simulink model "final_test2"  (Simulink 7.7)
settings: Solver=ode45  StartTime=0.0  StopTime=10.0  RelTol=1e-3
undefined symbols (not defined in the file): des_attributefunction_support, des_figposition
libraries: simeventsattributes2 x84, simeventsrouting1 x60, simeventsserver1 x31, commrandsrc2 x24, simeventsgenerators1 x16, simeventstranslate1 x15, simeventssink1 x12, simeventsqueue1 x8
(part 2 of 3)

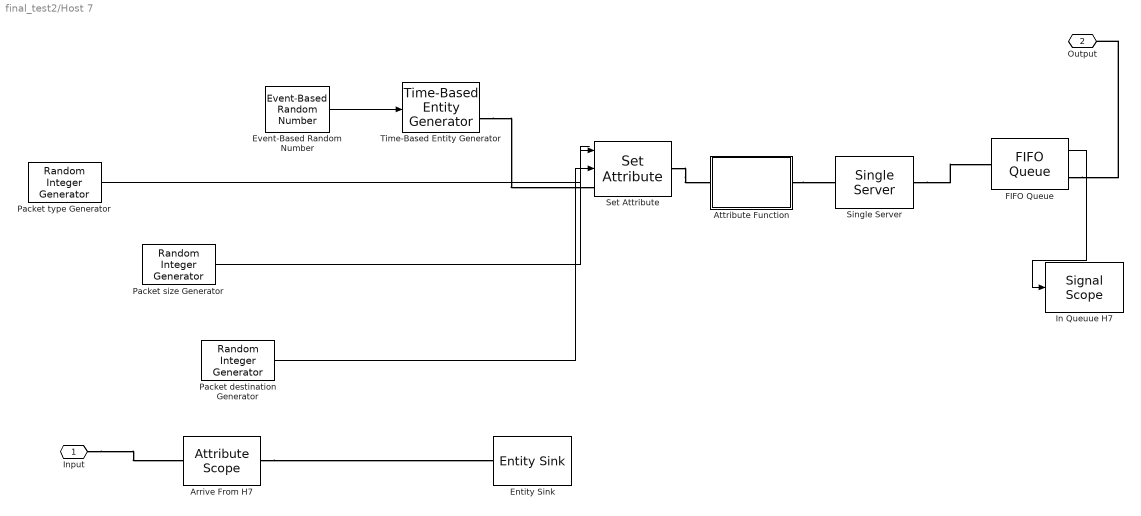
== system final_test2/Host 7 ==
  Arrive From H7 : simeventssink1/Attribute Scope  SystemSampleTime=-1  PlotType=Stair  InputType=Attribute  NumInputs=1  AttributeNameY=from  XInputOptionSignal=Event time  XInputOptionEntity=Event time  AttributeNameX=Count  EnableEntityOutport=on  XMin=0  XMax=10  XLimitExceededOption=Stretch axis limits  YLimitExceededOption=Stretch axis limits  AxisGrid=on  AxisLegend=off  LineDisables=""  LineColors=b  LineStyles=-  LineMarkers=.  OpenScopeAtSimStart=on  Title=""  YLabel=""  XLabel=Time  FigurePosition=des_figposition([5 25 25 25])  AxisZoom=off  DataStoreOption=Limited  DataPointsLimit=10000  StatNumberArrived=Off  ShowCountPlotted=off  ShowToolbar=on
      settings: YMin=0  YMax=10
  Attribute Function : Subsystem  LoadFcn=des_attributefunction_support(gcb,'LoadFcn');  StartFcn=des_attributefunction_support(gcb,'StartFcn');  mask(Attribute Function){OutputNamePrefix=out_}
      mask prompts: OutputNamePrefix "Prefix name"
      settings: CopyFcn=des_attributefunction_support(gcb,'CopyFcn');  OpenFcn=des_attributefunction_support(gcb,'OpenFcn');  ErrorFcn=des_error_redirect
      mask Help: helpview(simeventsbhelp('attributefunction'))
      mask Display: image(des_iconLoad('attribFunction.jpg'),'center');
  Entity Sink : simeventssink1/Entity Sink  SystemSampleTime=-1  AvailableForArrivals=on  StatNumberArrived=On
  Event-Based Random Number : simeventsgenerators1/Signal Generators/Event-Based Random Number  SystemSampleTime=-1  distribution=Poisson  meanExp=1  minUnif=1  maxUnif=1  pOneBern=0.25  pSuccessBino=0.5  numTrialBino=1  meanNorm=0  stdNorm=1  minTri=1  maxTri=3  modeTri=2  thresholdLogn=0  scaleLogn=1  shapeLogn=1  pSuccessGeo=0.5  meanPoiss=0.001  thresholdLogl=0  scaleLogl=1  thresholdGam=0  scaleGam=1  shapeGam=1  minBeta=0  maxBeta=1  shape1Beta=1  shape2Beta=1  minUnid=0  maxUnid=1  numValueUnid=2  thresholdWbl=0  scaleWbl=1  shapeWbl=1  valueVecCont=[0 1]  cdfVecCont=[0 1]  valueVecDisc=[0 1]  probVecDisc=[0.5 0.5]  seed=12345  IsProcessed=on  isConnected=1
  FIFO Queue : simeventsqueue1/FIFO Queue  SystemSampleTime=-1  Capacity=25  EnableTOPort=off  StatNumberDeparted=Off  StatNumberInBlock=On  StatPendingEntity=Off  StatAverageWait=Off  StatAverageQueueLength=Off  StatNumberTimedout=Off
  In Queuue H7 : simeventssink1/Signal Scope  SystemSampleTime=-1  PlotType=Stair  InputType=Signal  NumInputs=1  AttributeNameY=Count  XInputOptionSignal=Event time  XInputOptionEntity=Event time  AttributeNameX=Count  EnableEntityOutport=on  XMin=0  XMax=10  XLimitExceededOption=Stretch axis limits  YLimitExceededOption=Stretch axis limits  AxisGrid=on  AxisLegend=off  LineDisables=""  LineColors=b  LineStyles=-  LineMarkers=.  OpenScopeAtSimStart=on  Title=""  YLabel=""  XLabel=Time  FigurePosition=des_figposition([5 60 25 25])  AxisZoom=off  DataStoreOption=Limited  DataPointsLimit=10000  StatNumberArrived=Off  ShowCountPlotted=off  ShowToolbar=on
      settings: YMin=0  YMax=10
  Packet destination Generator : commrandsrc2/Random Integer Generator  SystemSampleTime=-1  mul=6  seed=22  Ts=1  frameBased=off  sampPerFrame=1  orient=off  outDataType=double
  Packet size Generator : commrandsrc2/Random Integer Generator  SystemSampleTime=-1  mul=2  seed=22  Ts=1  frameBased=off  sampPerFrame=1  orient=off  outDataType=double
  Packet type Generator : commrandsrc2/Random Integer Generator  SystemSampleTime=-1  mul=2  seed=37  Ts=1  frameBased=off  sampPerFrame=1  orient=off  outDataType=double
  Set Attribute : simeventsattributes2/Set Attribute  SystemSampleTime=-1  AttributeFrom=Dialog|Signal port|Signal port|Dialog  AttributeName=type|size|dest|from  AttributeTreatAsVector=1|1|1|1  AttributeValue=1|1|4|1  AttributeCreate=on  StatNumberDeparted=Off  EvaluatedAttributeValue={1;[];[];1}
  Single Server : simeventsserver1/Single Server  SystemSampleTime=-1  ServiceTimeFrom=Dialog  ServiceTime=0  AttributeName=ServiceTime  PriorityServiceCompletion=500  PermitPreemption=off  SortingAttributeName=PriorityAttributeName  SortingDirection=Ascending  WriteToAttribute=off  ResidualAttributeName=ResidualServiceTime  CreateAttribute=on  EnableTOPort=off  StatNumberDeparted=Off  StatNumberInBlock=Off  StatNumberPreempted=Off  StatPendingEntity=Off  StatAverageWait=Off  StatUtilization=Off  StatNumberTimedout=Off
  Time-Based Entity Generator : simeventsgenerators1/Entity Generators/Time-Based Entity Generator  SystemSampleTime=-1  GenerateEntitiesUpon=Intergeneration time from port t  Distribution=Constant  Minimum=0  Maximum=1  Mean=1  InitialSeed=12345  Period=1  PriorityEntityGeneration=300  GenerateEntityAtSimulationStart=on  ResponseWhenBlocked=Pause generation  ResponseWhenUnblocked=Immediate restart  EntityType=Standard  StatNumberDeparted=On  StatPendingEntity=Off  StatAverageIntergenerationTime=Off
  Input : PMIOPort  Port=1  Side=Right
  Output : PMIOPort  Port=2  Side=Right
  wires:
  Event-Based Random Number/1 -> Time-Based Entity Generator/1
  Packet size Generator/1 -> Set Attribute/1
  Packet type Generator/1 -> ?
  Packet destination Generator/1 -> Set Attribute/2
  FIFO Queue/1 -> In Queuue H7/1
  connections:
  Time-Based Entity Generator/RConn1 -- Set Attribute/LConn1
  Set Attribute/RConn1 -- Attribute Function/LConn1
  FIFO Queue/RConn1 -- Output/RConn1
  Attribute Function/RConn1 -- Single Server/LConn1
  Single Server/RConn1 -- FIFO Queue/LConn1
  Input/RConn1 -- Arrive From H7/LConn1
  Arrive From H7/RConn1 -- Entity Sink/LConn1

== system final_test2/Host 8 ==
  Attribute Function : Subsystem  LoadFcn=des_attributefunction_support(gcb,'LoadFcn');  StartFcn=des_attributefunction_support(gcb,'StartFcn');  mask(Attribute Function){OutputNamePrefix=out_}
      mask prompts: OutputNamePrefix "Prefix name"
      settings: CopyFcn=des_attributefunction_support(gcb,'CopyFcn');  OpenFcn=des_attributefunction_support(gcb,'OpenFcn');  ErrorFcn=des_error_redirect
      mask Help: helpview(simeventsbhelp('attributefunction'))
      mask Display: image(des_iconLoad('attribFunction.jpg'),'center');
  Entity Sink : simeventssink1/Entity Sink  SystemSampleTime=-1  AvailableForArrivals=on  StatNumberArrived=On
  Event-Based Random Number : simeventsgenerators1/Signal Generators/Event-Based Random Number  SystemSampleTime=-1  distribution=Poisson  meanExp=1  minUnif=1  maxUnif=1  pOneBern=0.25  pSuccessBino=0.5  numTrialBino=1  meanNorm=0  stdNorm=1  minTri=1  maxTri=3  modeTri=2  thresholdLogn=0  scaleLogn=1  shapeLogn=1  pSuccessGeo=0.5  meanPoiss=0.1  thresholdLogl=0  scaleLogl=1  thresholdGam=0  scaleGam=1  shapeGam=1  minBeta=0  maxBeta=1  shape1Beta=1  shape2Beta=1  minUnid=0  maxUnid=1  numValueUnid=2  thresholdWbl=0  scaleWbl=1  shapeWbl=1  valueVecCont=[0 1]  cdfVecCont=[0 1]  valueVecDisc=[0 1]  probVecDisc=[0.5 0.5]  seed=12345  IsProcessed=on  isConnected=1
  FIFO Queue : simeventsqueue1/FIFO Queue  SystemSampleTime=-1  Capacity=25  EnableTOPort=off  StatNumberDeparted=Off  StatNumberInBlock=Off  StatPendingEntity=Off  StatAverageWait=Off  StatAverageQueueLength=Off  StatNumberTimedout=Off
  Packet destination Generator : commrandsrc2/Random Integer Generator  SystemSampleTime=-1  mul=6  seed=22  Ts=1  frameBased=off  sampPerFrame=1  orient=off  outDataType=double
  Packet size Generator : commrandsrc2/Random Integer Generator  SystemSampleTime=-1  mul=2  seed=22  Ts=1  frameBased=off  sampPerFrame=1  orient=off  outDataType=double
  Packet type Generator : commrandsrc2/Random Integer Generator  SystemSampleTime=-1  mul=2  seed=37  Ts=1  frameBased=off  sampPerFrame=1  orient=off  outDataType=double
  Set Attribute : simeventsattributes2/Set Attribute  SystemSampleTime=-1  AttributeFrom=Signal port|Signal port|Signal port|Dialog  AttributeName=type|size|dest|from  AttributeTreatAsVector=1|1|1|1  AttributeValue=1|1|4|6  AttributeCreate=on  StatNumberDeparted=Off  EvaluatedAttributeValue={[];[];[];6}
  Single Server : simeventsserver1/Single Server  SystemSampleTime=-1  ServiceTimeFrom=Dialog  ServiceTime=0  AttributeName=ServiceTime  PriorityServiceCompletion=500  PermitPreemption=off  SortingAttributeName=PriorityAttributeName  SortingDirection=Ascending  WriteToAttribute=off  ResidualAttributeName=ResidualServiceTime  CreateAttribute=on  EnableTOPort=off  StatNumberDeparted=Off  StatNumberInBlock=Off  StatNumberPreempted=Off  StatPendingEntity=Off  StatAverageWait=Off  StatUtilization=Off  StatNumberTimedout=Off
  Time-Based Entity Generator : simeventsgenerators1/Entity Generators/Time-Based Entity Generator  SystemSampleTime=-1  GenerateEntitiesUpon=Intergeneration time from port t  Distribution=Constant  Minimum=0  Maximum=1  Mean=1  InitialSeed=12345  Period=1  PriorityEntityGeneration=300  GenerateEntityAtSimulationStart=on  ResponseWhenBlocked=Pause generation  ResponseWhenUnblocked=Immediate restart  EntityType=Standard  StatNumberDeparted=On  StatPendingEntity=Off  StatAverageIntergenerationTime=Off
  Input : PMIOPort  Port=1  Side=Left
  Output : PMIOPort  Port=2  Side=Left
  wires:
  Packet destination Generator/1 -> Set Attribute/3
  Packet type Generator/1 -> Set Attribute/1
  Packet size Generator/1 -> Set Attribute/2
  Event-Based Random Number/1 -> Time-Based Entity Generator/1
  connections:
  Single Server/RConn1 -- FIFO Queue/LConn1
  Attribute Function/RConn1 -- Single Server/LConn1
  FIFO Queue/RConn1 -- Output/RConn1
  Set Attribute/RConn1 -- Attribute Function/LConn1
  Input/RConn1 -- Entity Sink/LConn1
  Time-Based Entity Generator/RConn1 -- Set Attribute/LConn1

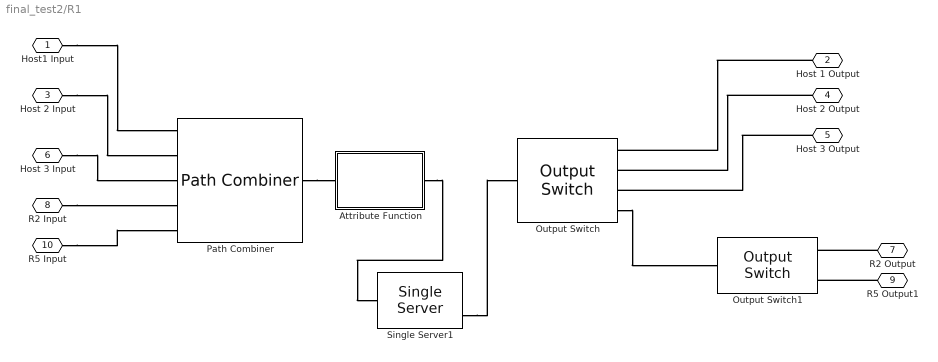
== system final_test2/R1 ==
  Attribute Function : Subsystem  LoadFcn=des_attributefunction_support(gcb,'LoadFcn');  StartFcn=des_attributefunction_support(gcb,'StartFcn');  mask(Attribute Function){OutputNamePrefix=out_}
      mask prompts: OutputNamePrefix "Prefix name"
      settings: CopyFcn=des_attributefunction_support(gcb,'CopyFcn');  OpenFcn=des_attributefunction_support(gcb,'OpenFcn');  ErrorFcn=des_error_redirect
      mask Help: helpview(simeventsbhelp('attributefunction'))
      mask Display: image(des_iconLoad('attribFunction.jpg'),'center');
  Output Switch : simeventsrouting1/Output Switch  SystemSampleTime=-1  NumberOutputPorts=4  SwitchingCriterion=From attribute  InitialSeed=34567  AttributeName=port  InitialConditionsOpt=off  InitialConditions=1  EntityBufferOpt=off  SpecifyEventPriority=off  PriorityOutputSwitchSelectPort=4100  TimeoutPortOpt=off  StatNumberDeparted=Off  StatNumberTimedOut=Off  StatPendingEntity=Off  StatLastDeparturePort=Off  EvaluatedNumPorts=4
  Output Switch1 : simeventsrouting1/Output Switch  SystemSampleTime=-1  NumberOutputPorts=2  SwitchingCriterion=First port that is not blocked  InitialSeed=34567  AttributeName=Attribute1  InitialConditionsOpt=off  InitialConditions=1  EntityBufferOpt=off  SpecifyEventPriority=off  PriorityOutputSwitchSelectPort=4100  TimeoutPortOpt=off  StatNumberDeparted=Off  StatNumberTimedOut=Off  StatPendingEntity=Off  StatLastDeparturePort=Off  EvaluatedNumPorts=2
  Path Combiner : simeventsrouting1/Path Combiner  SystemSampleTime=-1  NumberInputPorts=5  InputPortPrecedence=IN1 port  InitialSeed=45675  SpecifyEventPriority=off  PriorityPathCombinerPortPrecedenceSelection=4100  StatNumberDeparted=Off  StatLastArrivalPort=Off  EvaluatedNumPorts=5
  Single Server1 : simeventsserver1/Single Server  SystemSampleTime=-1  ServiceTimeFrom=Dialog  ServiceTime=0  AttributeName=ServiceTime  PriorityServiceCompletion=500  PermitPreemption=off  SortingAttributeName=PriorityAttributeName  SortingDirection=Ascending  WriteToAttribute=off  ResidualAttributeName=ResidualServiceTime  CreateAttribute=on  EnableTOPort=off  StatNumberDeparted=On  StatNumberInBlock=Off  StatNumberPreempted=Off  StatPendingEntity=Off  StatAverageWait=Off  StatUtilization=Off  StatNumberTimedout=Off
  Host1 Input : PMIOPort  Port=1  Side=Left
  Host 1 Output : PMIOPort  Port=2  Side=Left
  Host 2 Input : PMIOPort  Port=3  Side=Left
  Host 2 Output : PMIOPort  Port=4  Side=Left
  Host 3 Output : PMIOPort  Port=5  Side=Left
  Host 3 Input : PMIOPort  Port=6  Side=Left
  R2 Output : PMIOPort  Port=7  Side=Right
  R2 Input : PMIOPort  Port=8  Side=Right
  R5 Output1 : PMIOPort  Port=9  Side=Right
  R5 Input : PMIOPort  Port=10  Side=Right
  connections:
  Host 1 Output/RConn1 -- Output Switch/RConn1
  Host 2 Output/RConn1 -- Output Switch/RConn2
  Host 3 Output/RConn1 -- Output Switch/RConn3
  Host1 Input/RConn1 -- Path Combiner/LConn1
  Host 2 Input/RConn1 -- Path Combiner/LConn2
  Host 3 Input/RConn1 -- Path Combiner/LConn3
  R2 Input/RConn1 -- Path Combiner/LConn4
  R5 Input/RConn1 -- Path Combiner/LConn5
  Output Switch/RConn4 -- Output Switch1/LConn1
  R2 Output/RConn1 -- Output Switch1/RConn1
  R5 Output1/RConn1 -- Output Switch1/RConn2
  Path Combiner/RConn1 -- Attribute Function/LConn1
  Attribute Function/RConn1 -- Single Server1/LConn1
  Single Server1/RConn1 -- Output Switch/LConn1

== system final_test2/R2 ==
  Attribute Function : Subsystem  LoadFcn=des_attributefunction_support(gcb,'LoadFcn');  StartFcn=des_attributefunction_support(gcb,'StartFcn');  mask(Attribute Function){OutputNamePrefix=out_}
      mask prompts: OutputNamePrefix "Prefix name"
      settings: CopyFcn=des_attributefunction_support(gcb,'CopyFcn');  OpenFcn=des_attributefunction_support(gcb,'OpenFcn');  ErrorFcn=des_error_redirect
      mask Help: helpview(simeventsbhelp('attributefunction'))
      mask Display: image(des_iconLoad('attribFunction.jpg'),'center');
  Output Switch : simeventsrouting1/Output Switch  SystemSampleTime=-1  NumberOutputPorts=2  SwitchingCriterion=From attribute  InitialSeed=34567  AttributeName=port  InitialConditionsOpt=off  InitialConditions=1  EntityBufferOpt=off  SpecifyEventPriority=off  PriorityOutputSwitchSelectPort=4100  TimeoutPortOpt=off  StatNumberDeparted=Off  StatNumberTimedOut=Off  StatPendingEntity=Off  StatLastDeparturePort=Off  EvaluatedNumPorts=2
  Path Combiner : simeventsrouting1/Path Combiner  SystemSampleTime=-1  NumberInputPorts=2  InputPortPrecedence=IN1 port  InitialSeed=45675  SpecifyEventPriority=off  PriorityPathCombinerPortPrecedenceSelection=4100  StatNumberDeparted=Off  StatLastArrivalPort=Off  EvaluatedNumPorts=2
  Set Attribute : simeventsattributes2/Set Attribute  SystemSampleTime=-1  AttributeFrom=Dialog  AttributeName=rfrom  AttributeTreatAsVector=1  AttributeValue=1  AttributeCreate=on  StatNumberDeparted=Off  EvaluatedAttributeValue={1}
  Set Attribute1 : simeventsattributes2/Set Attribute  SystemSampleTime=-1  AttributeFrom=Dialog  AttributeName=rfrom  AttributeTreatAsVector=1  AttributeValue=3  AttributeCreate=on  StatNumberDeparted=Off  EvaluatedAttributeValue={3}
  Single Server : simeventsserver1/Single Server  SystemSampleTime=-1  ServiceTimeFrom=Dialog  ServiceTime=0  AttributeName=ServiceTime  PriorityServiceCompletion=500  PermitPreemption=off  SortingAttributeName=PriorityAttributeName  SortingDirection=Ascending  WriteToAttribute=off  ResidualAttributeName=ResidualServiceTime  CreateAttribute=on  EnableTOPort=off  StatNumberDeparted=Off  StatNumberInBlock=Off  StatNumberPreempted=Off  StatPendingEntity=Off  StatAverageWait=Off  StatUtilization=Off  StatNumberTimedout=Off
  R1 In : PMIOPort  Port=1  Side=Left
  R1 Out : PMIOPort  Port=2  Side=Left
  R3 Out : PMIOPort  Port=3  Side=Right
  R3 In : PMIOPort  Port=4  Side=Right
  connections:
  Path Combiner/RConn1 -- Attribute Function/LConn1
  Set Attribute/RConn1 -- Path Combiner/LConn1
  Set Attribute1/RConn1 -- Path Combiner/LConn2
  R1 In/RConn1 -- Set Attribute/LConn1
  R1 Out/RConn1 -- Output Switch/RConn1
  R3 Out/RConn1 -- Output Switch/RConn2
  R3 In/RConn1 -- Set Attribute1/LConn1
  Single Server/RConn1 -- Output Switch/LConn1
  Attribute Function/RConn1 -- Single Server/LConn1

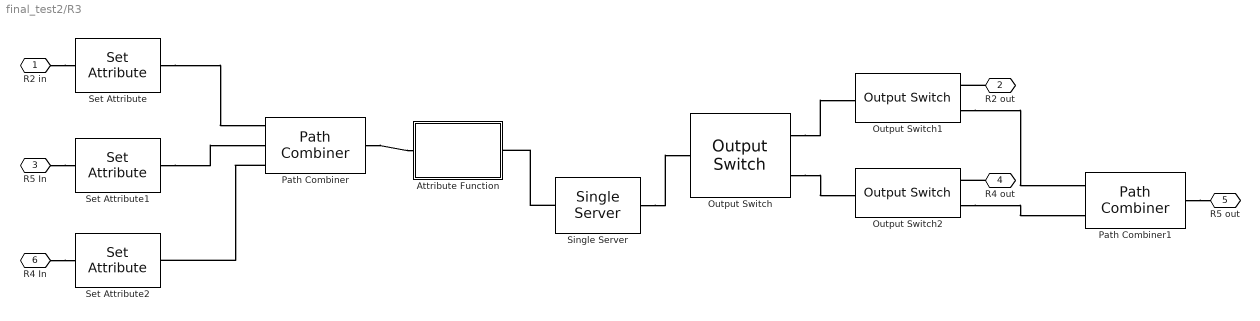
== system final_test2/R3 ==
  Attribute Function : Subsystem  LoadFcn=des_attributefunction_support(gcb,'LoadFcn');  StartFcn=des_attributefunction_support(gcb,'StartFcn');  mask(Attribute Function){OutputNamePrefix=out_}
      mask prompts: OutputNamePrefix "Prefix name"
      settings: CopyFcn=des_attributefunction_support(gcb,'CopyFcn');  OpenFcn=des_attributefunction_support(gcb,'OpenFcn');  ErrorFcn=des_error_redirect
      mask Help: helpview(simeventsbhelp('attributefunction'))
      mask Display: image(des_iconLoad('attribFunction.jpg'),'center');
  Output Switch : simeventsrouting1/Output Switch  SystemSampleTime=-1  NumberOutputPorts=2  SwitchingCriterion=From attribute  InitialSeed=34567  AttributeName=port  InitialConditionsOpt=off  InitialConditions=1  EntityBufferOpt=off  SpecifyEventPriority=off  PriorityOutputSwitchSelectPort=4100  TimeoutPortOpt=off  StatNumberDeparted=Off  StatNumberTimedOut=Off  StatPendingEntity=Off  StatLastDeparturePort=Off  EvaluatedNumPorts=2
  Output Switch1 : simeventsrouting1/Output Switch  SystemSampleTime=-1  NumberOutputPorts=2  SwitchingCriterion=First port that is not blocked  InitialSeed=34567  AttributeName=port  InitialConditionsOpt=off  InitialConditions=1  EntityBufferOpt=off  SpecifyEventPriority=off  PriorityOutputSwitchSelectPort=4100  TimeoutPortOpt=off  StatNumberDeparted=Off  StatNumberTimedOut=Off  StatPendingEntity=Off  StatLastDeparturePort=Off  EvaluatedNumPorts=2
  Output Switch2 : simeventsrouting1/Output Switch  SystemSampleTime=-1  NumberOutputPorts=2  SwitchingCriterion=First port that is not blocked  InitialSeed=34567  AttributeName=port  InitialConditionsOpt=off  InitialConditions=1  EntityBufferOpt=off  SpecifyEventPriority=off  PriorityOutputSwitchSelectPort=4100  TimeoutPortOpt=off  StatNumberDeparted=Off  StatNumberTimedOut=Off  StatPendingEntity=Off  StatLastDeparturePort=Off  EvaluatedNumPorts=2
  Path Combiner : simeventsrouting1/Path Combiner  SystemSampleTime=-1  NumberInputPorts=3  InputPortPrecedence=IN1 port  InitialSeed=45675  SpecifyEventPriority=off  PriorityPathCombinerPortPrecedenceSelection=4100  StatNumberDeparted=Off  StatLastArrivalPort=Off  EvaluatedNumPorts=3
  Path Combiner1 : simeventsrouting1/Path Combiner  SystemSampleTime=-1  NumberInputPorts=2  InputPortPrecedence=IN1 port  InitialSeed=45675  SpecifyEventPriority=off  PriorityPathCombinerPortPrecedenceSelection=4100  StatNumberDeparted=Off  StatLastArrivalPort=Off  EvaluatedNumPorts=2
  Set Attribute : simeventsattributes2/Set Attribute  SystemSampleTime=-1  AttributeFrom=Dialog  AttributeName=rfrom  AttributeTreatAsVector=1  AttributeValue=2  AttributeCreate=on  StatNumberDeparted=Off  EvaluatedAttributeValue={2}
  Set Attribute1 : simeventsattributes2/Set Attribute  SystemSampleTime=-1  AttributeFrom=Dialog  AttributeName=rfrom  AttributeTreatAsVector=1  AttributeValue=5  AttributeCreate=on  StatNumberDeparted=Off  EvaluatedAttributeValue={5}
  Set Attribute2 : simeventsattributes2/Set Attribute  SystemSampleTime=-1  AttributeFrom=Dialog  AttributeName=rfrom  AttributeTreatAsVector=1  AttributeValue=4  AttributeCreate=on  StatNumberDeparted=Off  EvaluatedAttributeValue={4}
  Single Server : simeventsserver1/Single Server  SystemSampleTime=-1  ServiceTimeFrom=Dialog  ServiceTime=0  AttributeName=ServiceTime  PriorityServiceCompletion=500  PermitPreemption=off  SortingAttributeName=PriorityAttributeName  SortingDirection=Ascending  WriteToAttribute=off  ResidualAttributeName=ResidualServiceTime  CreateAttribute=on  EnableTOPort=off  StatNumberDeparted=Off  StatNumberInBlock=Off  StatNumberPreempted=Off  StatPendingEntity=Off  StatAverageWait=Off  StatUtilization=Off  StatNumberTimedout=Off
  R2 in : PMIOPort  Port=1  Side=Left
  R2 out : PMIOPort  Port=2  Side=Left
  R5 In : PMIOPort  Port=3  Side=Left
  R4 out : PMIOPort  Port=4  Side=Right
  R5 out : PMIOPort  Port=5  Side=Left
  R4 In : PMIOPort  Port=6  Side=Right
  connections:
  Path Combiner/RConn1 -- Attribute Function/LConn1
  Output Switch/RConn1 -- Output Switch1/LConn1
  Output Switch/RConn2 -- Output Switch2/LConn1
  Set Attribute/RConn1 -- Path Combiner/LConn1
  Set Attribute1/RConn1 -- Path Combiner/LConn2
  Path Combiner/LConn3 -- Set Attribute2/RConn1
  R2 in/RConn1 -- Set Attribute/LConn1
  R2 out/RConn1 -- Output Switch1/RConn1
  R5 In/RConn1 -- Set Attribute1/LConn1
  R4 out/RConn1 -- Output Switch2/RConn1
  R4 In/RConn1 -- Set Attribute2/LConn1
  Path Combiner1/RConn1 -- R5 out/RConn1
  Output Switch2/RConn2 -- Path Combiner1/LConn2
  Output Switch1/RConn2 -- Path Combiner1/LConn1
  Single Server/RConn1 -- Output Switch/LConn1
  Single Server/LConn1 -- Attribute Function/RConn1

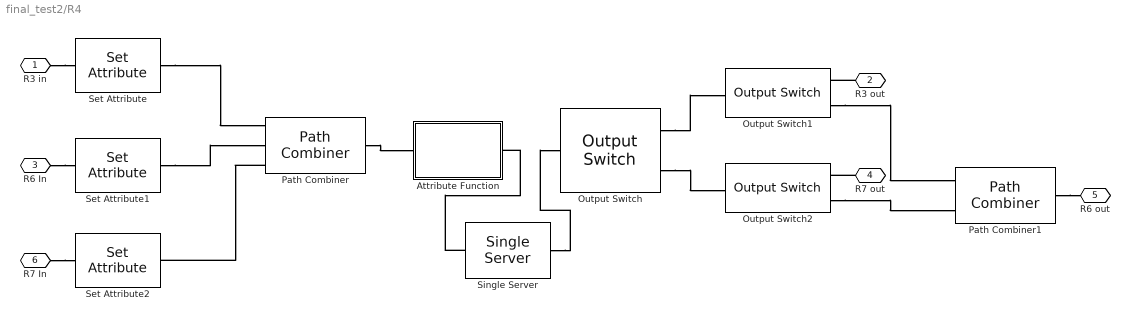
== system final_test2/R4 ==
  Attribute Function : Subsystem  LoadFcn=des_attributefunction_support(gcb,'LoadFcn');  StartFcn=des_attributefunction_support(gcb,'StartFcn');  mask(Attribute Function){OutputNamePrefix=out_}
      mask prompts: OutputNamePrefix "Prefix name"
      settings: CopyFcn=des_attributefunction_support(gcb,'CopyFcn');  OpenFcn=des_attributefunction_support(gcb,'OpenFcn');  ErrorFcn=des_error_redirect
      mask Help: helpview(simeventsbhelp('attributefunction'))
      mask Display: image(des_iconLoad('attribFunction.jpg'),'center');
  Output Switch : simeventsrouting1/Output Switch  SystemSampleTime=-1  NumberOutputPorts=2  SwitchingCriterion=From attribute  InitialSeed=34567  AttributeName=port  InitialConditionsOpt=off  InitialConditions=1  EntityBufferOpt=off  SpecifyEventPriority=off  PriorityOutputSwitchSelectPort=4100  TimeoutPortOpt=off  StatNumberDeparted=Off  StatNumberTimedOut=Off  StatPendingEntity=Off  StatLastDeparturePort=Off  EvaluatedNumPorts=2
  Output Switch1 : simeventsrouting1/Output Switch  SystemSampleTime=-1  NumberOutputPorts=2  SwitchingCriterion=First port that is not blocked  InitialSeed=34567  AttributeName=port  InitialConditionsOpt=off  InitialConditions=1  EntityBufferOpt=off  SpecifyEventPriority=off  PriorityOutputSwitchSelectPort=4100  TimeoutPortOpt=off  StatNumberDeparted=Off  StatNumberTimedOut=Off  StatPendingEntity=Off  StatLastDeparturePort=Off  EvaluatedNumPorts=2
  Output Switch2 : simeventsrouting1/Output Switch  SystemSampleTime=-1  NumberOutputPorts=2  SwitchingCriterion=First port that is not blocked  InitialSeed=34567  AttributeName=port  InitialConditionsOpt=off  InitialConditions=1  EntityBufferOpt=off  SpecifyEventPriority=off  PriorityOutputSwitchSelectPort=4100  TimeoutPortOpt=off  StatNumberDeparted=Off  StatNumberTimedOut=Off  StatPendingEntity=Off  StatLastDeparturePort=Off  EvaluatedNumPorts=2
  Path Combiner : simeventsrouting1/Path Combiner  SystemSampleTime=-1  NumberInputPorts=3  InputPortPrecedence=IN1 port  InitialSeed=45675  SpecifyEventPriority=off  PriorityPathCombinerPortPrecedenceSelection=4100  StatNumberDeparted=Off  StatLastArrivalPort=Off  EvaluatedNumPorts=3
  Path Combiner1 : simeventsrouting1/Path Combiner  SystemSampleTime=-1  NumberInputPorts=2  InputPortPrecedence=IN1 port  InitialSeed=45675  SpecifyEventPriority=off  PriorityPathCombinerPortPrecedenceSelection=4100  StatNumberDeparted=Off  StatLastArrivalPort=Off  EvaluatedNumPorts=2
  Set Attribute : simeventsattributes2/Set Attribute  SystemSampleTime=-1  AttributeFrom=Dialog  AttributeName=rfrom  AttributeTreatAsVector=1  AttributeValue=3  AttributeCreate=on  StatNumberDeparted=Off  EvaluatedAttributeValue={3}
  Set Attribute1 : simeventsattributes2/Set Attribute  SystemSampleTime=-1  AttributeFrom=Dialog  AttributeName=rfrom  AttributeTreatAsVector=1  AttributeValue=6  AttributeCreate=on  StatNumberDeparted=Off  EvaluatedAttributeValue={6}
  Set Attribute2 : simeventsattributes2/Set Attribute  SystemSampleTime=-1  AttributeFrom=Dialog  AttributeName=rfrom  AttributeTreatAsVector=1  AttributeValue=7  AttributeCreate=on  StatNumberDeparted=Off  EvaluatedAttributeValue={7}
  Single Server : simeventsserver1/Single Server  SystemSampleTime=-1  ServiceTimeFrom=Dialog  ServiceTime=0  AttributeName=ServiceTime  PriorityServiceCompletion=500  PermitPreemption=off  SortingAttributeName=PriorityAttributeName  SortingDirection=Ascending  WriteToAttribute=off  ResidualAttributeName=ResidualServiceTime  CreateAttribute=on  EnableTOPort=off  StatNumberDeparted=Off  StatNumberInBlock=Off  StatNumberPreempted=Off  StatPendingEntity=Off  StatAverageWait=Off  StatUtilization=Off  StatNumberTimedout=Off
  R3 in : PMIOPort  Port=1  Side=Left
  R3 out : PMIOPort  Port=2  Side=Left
  R6 In : PMIOPort  Port=3  Side=Left
  R7 out : PMIOPort  Port=4  Side=Right
  R6 out : PMIOPort  Port=5  Side=Left
  R7 In : PMIOPort  Port=6  Side=Right
  connections:
  Output Switch1/RConn2 -- Path Combiner1/LConn1
  Output Switch2/RConn2 -- Path Combiner1/LConn2
  Path Combiner1/RConn1 -- R6 out/RConn1
  R7 In/RConn1 -- Set Attribute2/LConn1
  R7 out/RConn1 -- Output Switch2/RConn1
  R6 In/RConn1 -- Set Attribute1/LConn1
  R3 out/RConn1 -- Output Switch1/RConn1
  R3 in/RConn1 -- Set Attribute/LConn1
  Path Combiner/LConn3 -- Set Attribute2/RConn1
  Set Attribute1/RConn1 -- Path Combiner/LConn2
  Set Attribute/RConn1 -- Path Combiner/LConn1
  Output Switch/RConn2 -- Output Switch2/LConn1
  Output Switch/RConn1 -- Output Switch1/LConn1
  Path Combiner/RConn1 -- Attribute Function/LConn1
  Single Server/LConn1 -- Attribute Function/RConn1
  Single Server/RConn1 -- Output Switch/LConn1

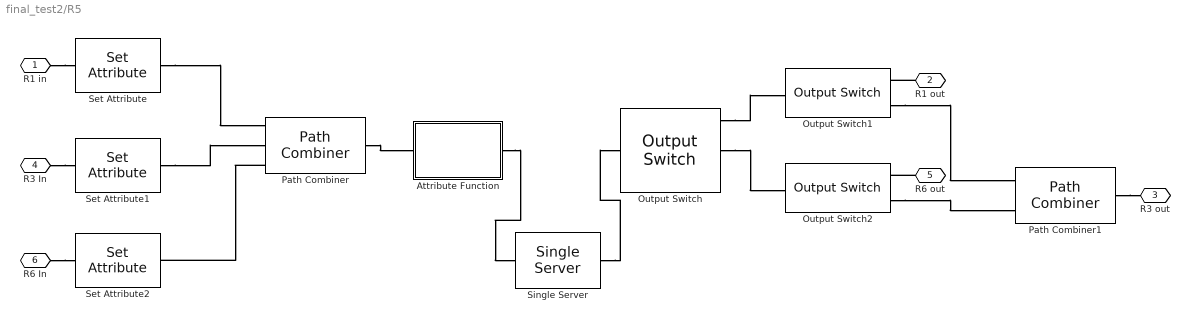
== system final_test2/R5 ==
  Attribute Function : Subsystem  LoadFcn=des_attributefunction_support(gcb,'LoadFcn');  StartFcn=des_attributefunction_support(gcb,'StartFcn');  mask(Attribute Function){OutputNamePrefix=out_}
      mask prompts: OutputNamePrefix "Prefix name"
      settings: CopyFcn=des_attributefunction_support(gcb,'CopyFcn');  OpenFcn=des_attributefunction_support(gcb,'OpenFcn');  ErrorFcn=des_error_redirect
      mask Help: helpview(simeventsbhelp('attributefunction'))
      mask Display: image(des_iconLoad('attribFunction.jpg'),'center');
  Output Switch : simeventsrouting1/Output Switch  SystemSampleTime=-1  NumberOutputPorts=3  SwitchingCriterion=From attribute  InitialSeed=34567  AttributeName=port  InitialConditionsOpt=off  InitialConditions=1  EntityBufferOpt=off  SpecifyEventPriority=off  PriorityOutputSwitchSelectPort=4100  TimeoutPortOpt=off  StatNumberDeparted=Off  StatNumberTimedOut=Off  StatPendingEntity=Off  StatLastDeparturePort=Off  EvaluatedNumPorts=3
  Output Switch1 : simeventsrouting1/Output Switch  SystemSampleTime=-1  NumberOutputPorts=2  SwitchingCriterion=First port that is not blocked  InitialSeed=34567  AttributeName=port  InitialConditionsOpt=off  InitialConditions=1  EntityBufferOpt=off  SpecifyEventPriority=off  PriorityOutputSwitchSelectPort=4100  TimeoutPortOpt=off  StatNumberDeparted=Off  StatNumberTimedOut=Off  StatPendingEntity=Off  StatLastDeparturePort=Off  EvaluatedNumPorts=2
  Output Switch2 : simeventsrouting1/Output Switch  SystemSampleTime=-1  NumberOutputPorts=2  SwitchingCriterion=First port that is not blocked  InitialSeed=34567  AttributeName=port  InitialConditionsOpt=off  InitialConditions=1  EntityBufferOpt=off  SpecifyEventPriority=off  PriorityOutputSwitchSelectPort=4100  TimeoutPortOpt=off  StatNumberDeparted=Off  StatNumberTimedOut=Off  StatPendingEntity=Off  StatLastDeparturePort=Off  EvaluatedNumPorts=2
  Path Combiner : simeventsrouting1/Path Combiner  SystemSampleTime=-1  NumberInputPorts=3  InputPortPrecedence=IN1 port  InitialSeed=45675  SpecifyEventPriority=off  PriorityPathCombinerPortPrecedenceSelection=4100  StatNumberDeparted=Off  StatLastArrivalPort=Off  EvaluatedNumPorts=3
  Path Combiner1 : simeventsrouting1/Path Combiner  SystemSampleTime=-1  NumberInputPorts=2  InputPortPrecedence=IN1 port  InitialSeed=45675  SpecifyEventPriority=off  PriorityPathCombinerPortPrecedenceSelection=4100  StatNumberDeparted=Off  StatLastArrivalPort=Off  EvaluatedNumPorts=2
  Set Attribute : simeventsattributes2/Set Attribute  SystemSampleTime=-1  AttributeFrom=Dialog  AttributeName=rfrom  AttributeTreatAsVector=1  AttributeValue=1  AttributeCreate=on  StatNumberDeparted=Off  EvaluatedAttributeValue={1}
  Set Attribute1 : simeventsattributes2/Set Attribute  SystemSampleTime=-1  AttributeFrom=Dialog  AttributeName=rfrom  AttributeTreatAsVector=1  AttributeValue=3  AttributeCreate=on  StatNumberDeparted=Off  EvaluatedAttributeValue={3}
  Set Attribute2 : simeventsattributes2/Set Attribute  SystemSampleTime=-1  AttributeFrom=Dialog  AttributeName=rfrom  AttributeTreatAsVector=1  AttributeValue=6  AttributeCreate=on  StatNumberDeparted=Off  EvaluatedAttributeValue={6}
  Single Server : simeventsserver1/Single Server  SystemSampleTime=-1  ServiceTimeFrom=Dialog  ServiceTime=0  AttributeName=ServiceTime  PriorityServiceCompletion=500  PermitPreemption=off  SortingAttributeName=PriorityAttributeName  SortingDirection=Ascending  WriteToAttribute=off  ResidualAttributeName=ResidualServiceTime  CreateAttribute=on  EnableTOPort=off  StatNumberDeparted=Off  StatNumberInBlock=Off  StatNumberPreempted=Off  StatPendingEntity=Off  StatAverageWait=Off  StatUtilization=Off  StatNumberTimedout=Off
  R1 in : PMIOPort  Port=1  Side=Left
  R1 out : PMIOPort  Port=2  Side=Left
  R3 out : PMIOPort  Port=3  Side=Right
  R3 In : PMIOPort  Port=4  Side=Right
  R6 out : PMIOPort  Port=5  Side=Right
  R6 In : PMIOPort  Port=6  Side=Right
  connections:
  Output Switch1/RConn2 -- Path Combiner1/LConn1
  Output Switch2/RConn2 -- Path Combiner1/LConn2
  Path Combiner1/RConn1 -- R3 out/RConn1
  R6 In/RConn1 -- Set Attribute2/LConn1
  R6 out/RConn1 -- Output Switch2/RConn1
  R3 In/RConn1 -- Set Attribute1/LConn1
  R1 out/RConn1 -- Output Switch1/RConn1
  R1 in/RConn1 -- Set Attribute/LConn1
  Path Combiner/LConn3 -- Set Attribute2/RConn1
  Set Attribute1/RConn1 -- Path Combiner/LConn2
  Set Attribute/RConn1 -- Path Combiner/LConn1
  Path Combiner/RConn1 -- Attribute Function/LConn1
  Output Switch/RConn1 -- Output Switch1/LConn1
  Output Switch/RConn2 -- Output Switch2/LConn1
  Attribute Function/RConn1 -- Single Server/LConn1
  Single Server/RConn1 -- Output Switch/LConn1

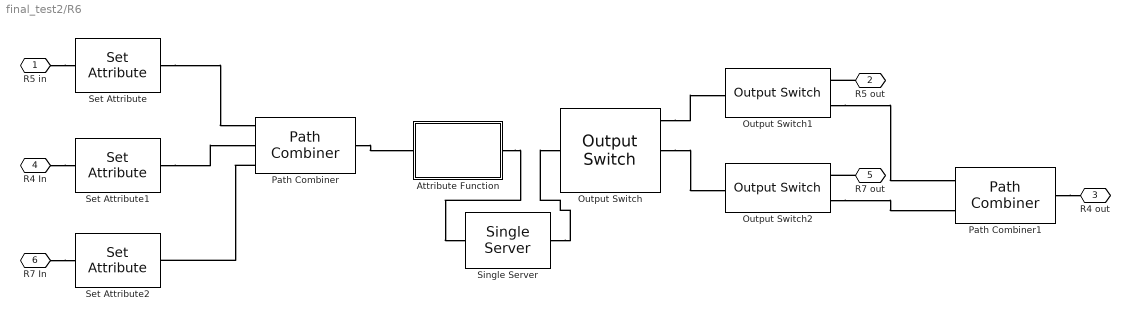
== system final_test2/R6 ==
  Attribute Function : Subsystem  LoadFcn=des_attributefunction_support(gcb,'LoadFcn');  StartFcn=des_attributefunction_support(gcb,'StartFcn');  mask(Attribute Function){OutputNamePrefix=out_}
      mask prompts: OutputNamePrefix "Prefix name"
      settings: CopyFcn=des_attributefunction_support(gcb,'CopyFcn');  OpenFcn=des_attributefunction_support(gcb,'OpenFcn');  ErrorFcn=des_error_redirect
      mask Help: helpview(simeventsbhelp('attributefunction'))
      mask Display: image(des_iconLoad('attribFunction.jpg'),'center');
  Output Switch : simeventsrouting1/Output Switch  SystemSampleTime=-1  NumberOutputPorts=3  SwitchingCriterion=From attribute  InitialSeed=34567  AttributeName=port  InitialConditionsOpt=off  InitialConditions=1  EntityBufferOpt=off  SpecifyEventPriority=off  PriorityOutputSwitchSelectPort=4100  TimeoutPortOpt=off  StatNumberDeparted=Off  StatNumberTimedOut=Off  StatPendingEntity=Off  StatLastDeparturePort=Off  EvaluatedNumPorts=3
  Output Switch1 : simeventsrouting1/Output Switch  SystemSampleTime=-1  NumberOutputPorts=2  SwitchingCriterion=First port that is not blocked  InitialSeed=34567  AttributeName=port  InitialConditionsOpt=off  InitialConditions=1  EntityBufferOpt=off  SpecifyEventPriority=off  PriorityOutputSwitchSelectPort=4100  TimeoutPortOpt=off  StatNumberDeparted=Off  StatNumberTimedOut=Off  StatPendingEntity=Off  StatLastDeparturePort=Off  EvaluatedNumPorts=2
  Output Switch2 : simeventsrouting1/Output Switch  SystemSampleTime=-1  NumberOutputPorts=2  SwitchingCriterion=First port that is not blocked  InitialSeed=34567  AttributeName=port  InitialConditionsOpt=off  InitialConditions=1  EntityBufferOpt=off  SpecifyEventPriority=off  PriorityOutputSwitchSelectPort=4100  TimeoutPortOpt=off  StatNumberDeparted=Off  StatNumberTimedOut=Off  StatPendingEntity=Off  StatLastDeparturePort=Off  EvaluatedNumPorts=2
  Path Combiner : simeventsrouting1/Path Combiner  SystemSampleTime=-1  NumberInputPorts=3  InputPortPrecedence=IN1 port  InitialSeed=45675  SpecifyEventPriority=off  PriorityPathCombinerPortPrecedenceSelection=4100  StatNumberDeparted=Off  StatLastArrivalPort=Off  EvaluatedNumPorts=3
  Path Combiner1 : simeventsrouting1/Path Combiner  SystemSampleTime=-1  NumberInputPorts=2  InputPortPrecedence=IN1 port  InitialSeed=45675  SpecifyEventPriority=off  PriorityPathCombinerPortPrecedenceSelection=4100  StatNumberDeparted=Off  StatLastArrivalPort=Off  EvaluatedNumPorts=2
  Set Attribute : simeventsattributes2/Set Attribute  SystemSampleTime=-1  AttributeFrom=Dialog  AttributeName=rfrom  AttributeTreatAsVector=1  AttributeValue=5  AttributeCreate=on  StatNumberDeparted=Off  EvaluatedAttributeValue={5}
  Set Attribute1 : simeventsattributes2/Set Attribute  SystemSampleTime=-1  AttributeFrom=Dialog  AttributeName=rfrom  AttributeTreatAsVector=1  AttributeValue=4  AttributeCreate=on  StatNumberDeparted=Off  EvaluatedAttributeValue={4}
  Set Attribute2 : simeventsattributes2/Set Attribute  SystemSampleTime=-1  AttributeFrom=Dialog  AttributeName=rfrom  AttributeTreatAsVector=1  AttributeValue=5  AttributeCreate=on  StatNumberDeparted=Off  EvaluatedAttributeValue={5}
  Single Server : simeventsserver1/Single Server  SystemSampleTime=-1  ServiceTimeFrom=Dialog  ServiceTime=0  AttributeName=ServiceTime  PriorityServiceCompletion=500  PermitPreemption=off  SortingAttributeName=PriorityAttributeName  SortingDirection=Ascending  WriteToAttribute=off  ResidualAttributeName=ResidualServiceTime  CreateAttribute=on  EnableTOPort=off  StatNumberDeparted=Off  StatNumberInBlock=Off  StatNumberPreempted=Off  StatPendingEntity=Off  StatAverageWait=Off  StatUtilization=Off  StatNumberTimedout=Off
  R5 in : PMIOPort  Port=1  Side=Left
  R5 out : PMIOPort  Port=2  Side=Left
  R4 out : PMIOPort  Port=3  Side=Right
  R4 In : PMIOPort  Port=4  Side=Right
  R7 out : PMIOPort  Port=5  Side=Right
  R7 In : PMIOPort  Port=6  Side=Right
  connections:
  Output Switch/RConn2 -- Output Switch2/LConn1
  Output Switch/RConn1 -- Output Switch1/LConn1
  Path Combiner/RConn1 -- Attribute Function/LConn1
  Set Attribute/RConn1 -- Path Combiner/LConn1
  Set Attribute1/RConn1 -- Path Combiner/LConn2
  Path Combiner/LConn3 -- Set Attribute2/RConn1
  R5 in/RConn1 -- Set Attribute/LConn1
  R5 out/RConn1 -- Output Switch1/RConn1
  R4 In/RConn1 -- Set Attribute1/LConn1
  R7 out/RConn1 -- Output Switch2/RConn1
  R7 In/RConn1 -- Set Attribute2/LConn1
  Path Combiner1/RConn1 -- R4 out/RConn1
  Output Switch2/RConn2 -- Path Combiner1/LConn2
  Output Switch1/RConn2 -- Path Combiner1/LConn1
  Attribute Function/RConn1 -- Single Server/LConn1
  Single Server/RConn1 -- Output Switch/LConn1

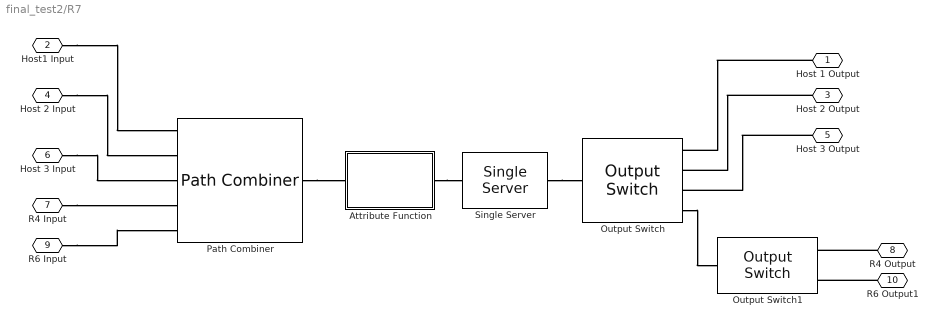
== system final_test2/R7 ==
  Attribute Function : Subsystem  LoadFcn=des_attributefunction_support(gcb,'LoadFcn');  StartFcn=des_attributefunction_support(gcb,'StartFcn');  mask(Attribute Function){OutputNamePrefix=out_}
      mask prompts: OutputNamePrefix "Prefix name"
      settings: CopyFcn=des_attributefunction_support(gcb,'CopyFcn');  OpenFcn=des_attributefunction_support(gcb,'OpenFcn');  ErrorFcn=des_error_redirect
      mask Help: helpview(simeventsbhelp('attributefunction'))
      mask Display: image(des_iconLoad('attribFunction.jpg'),'center');
  Output Switch : simeventsrouting1/Output Switch  SystemSampleTime=-1  NumberOutputPorts=4  SwitchingCriterion=From attribute  InitialSeed=34567  AttributeName=port  InitialConditionsOpt=off  InitialConditions=1  EntityBufferOpt=off  SpecifyEventPriority=off  PriorityOutputSwitchSelectPort=4100  TimeoutPortOpt=off  StatNumberDeparted=Off  StatNumberTimedOut=Off  StatPendingEntity=Off  StatLastDeparturePort=Off  EvaluatedNumPorts=4
  Output Switch1 : simeventsrouting1/Output Switch  SystemSampleTime=-1  NumberOutputPorts=2  SwitchingCriterion=First port that is not blocked  InitialSeed=34567  AttributeName=Attribute1  InitialConditionsOpt=off  InitialConditions=1  EntityBufferOpt=off  SpecifyEventPriority=off  PriorityOutputSwitchSelectPort=4100  TimeoutPortOpt=off  StatNumberDeparted=Off  StatNumberTimedOut=Off  StatPendingEntity=Off  StatLastDeparturePort=Off  EvaluatedNumPorts=2
  Path Combiner : simeventsrouting1/Path Combiner  SystemSampleTime=-1  NumberInputPorts=5  InputPortPrecedence=IN1 port  InitialSeed=45675  SpecifyEventPriority=off  PriorityPathCombinerPortPrecedenceSelection=4100  StatNumberDeparted=Off  StatLastArrivalPort=Off  EvaluatedNumPorts=5
  Single Server : simeventsserver1/Single Server  SystemSampleTime=-1  ServiceTimeFrom=Dialog  ServiceTime=0  AttributeName=ServiceTime  PriorityServiceCompletion=500  PermitPreemption=off  SortingAttributeName=PriorityAttributeName  SortingDirection=Ascending  WriteToAttribute=off  ResidualAttributeName=ResidualServiceTime  CreateAttribute=on  EnableTOPort=off  StatNumberDeparted=Off  StatNumberInBlock=Off  StatNumberPreempted=Off  StatPendingEntity=Off  StatAverageWait=Off  StatUtilization=Off  StatNumberTimedout=Off
  Host 1 Output : PMIOPort  Port=1  Side=Right
  Host1 Input : PMIOPort  Port=2  Side=Right
  Host 2 Output : PMIOPort  Port=3  Side=Right
  Host 2 Input : PMIOPort  Port=4  Side=Right
  Host 3 Output : PMIOPort  Port=5  Side=Right
  Host 3 Input : PMIOPort  Port=6  Side=Right
  R4 Input : PMIOPort  Port=7  Side=Left
  R4 Output : PMIOPort  Port=8  Side=Left
  R6 Input : PMIOPort  Port=9  Side=Left
  R6 Output1 : PMIOPort  Port=10  Side=Left
  connections:
  Single Server/RConn1 -- Output Switch/LConn1
  Attribute Function/RConn1 -- Single Server/LConn1
  R6 Output1/RConn1 -- Output Switch1/RConn2
  R4 Output/RConn1 -- Output Switch1/RConn1
  Output Switch/RConn4 -- Output Switch1/LConn1
  R6 Input/RConn1 -- Path Combiner/LConn5
  R4 Input/RConn1 -- Path Combiner/LConn4
  Host 3 Input/RConn1 -- Path Combiner/LConn3
  Host 2 Input/RConn1 -- Path Combiner/LConn2
  Host1 Input/RConn1 -- Path Combiner/LConn1
  Host 3 Output/RConn1 -- Output Switch/RConn3
  Host 2 Output/RConn1 -- Output Switch/RConn2
  Host 1 Output/RConn1 -- Output Switch/RConn1
  Path Combiner/RConn1 -- Attribute Function/LConn1

== system final_test2/Red Link ==
  N-Server : simeventsserver1/N-Server  SystemSampleTime=-1  NumberOfServers=2  ServiceTimeFrom=Dialog  ServiceTime=0.001  AttributeName=ServiceTime  PriorityServiceCompletion=500  EnableTOPort=off  StatNumberDeparted=Off  StatNumberInBlock=Off  StatPendingEntity=Off  StatNumberPending=Off  StatAverageWait=Off  StatUtilization=Off  StatNumberTimedout=Off
  Output Switch : simeventsrouting1/Output Switch  SystemSampleTime=-1  NumberOutputPorts=2  SwitchingCriterion=From attribute  InitialSeed=34567  AttributeName=port  InitialConditionsOpt=off  InitialConditions=1  EntityBufferOpt=off  SpecifyEventPriority=off  PriorityOutputSwitchSelectPort=4100  TimeoutPortOpt=off  StatNumberDeparted=Off  StatNumberTimedOut=Off  StatPendingEntity=Off  StatLastDeparturePort=Off  EvaluatedNumPorts=2
  Path Combiner : simeventsrouting1/Path Combiner  SystemSampleTime=-1  NumberInputPorts=2  InputPortPrecedence=IN1 port  InitialSeed=45675  SpecifyEventPriority=off  PriorityPathCombinerPortPrecedenceSelection=4100  StatNumberDeparted=Off  StatLastArrivalPort=Off  EvaluatedNumPorts=2
  Set Attribute : simeventsattributes2/Set Attribute  SystemSampleTime=-1  AttributeFrom=Dialog  AttributeName=port  AttributeTreatAsVector=1  AttributeValue=1  AttributeCreate=on  StatNumberDeparted=Off  EvaluatedAttributeValue={1}
  Set Attribute1 : simeventsattributes2/Set Attribute  SystemSampleTime=-1  AttributeFrom=Dialog  AttributeName=port  AttributeTreatAsVector=1  AttributeValue=2  AttributeCreate=on  StatNumberDeparted=Off  EvaluatedAttributeValue={2}
  Input1 : PMIOPort  Port=1  Side=Left
  Output1 : PMIOPort  Port=2  Side=Right
  Input2 : PMIOPort  Port=3  Side=Right
  Output2 : PMIOPort  Port=4  Side=Left
  connections:
  Path Combiner/RConn1 -- N-Server/LConn1
  N-Server/RConn1 -- Output Switch/LConn1
  Output Switch/RConn1 -- Output1/RConn1
  Output Switch/RConn2 -- Output2/RConn1
  Input1/RConn1 -- Set Attribute/LConn1
  Set Attribute/RConn1 -- Path Combiner/LConn1
  Input2/RConn1 -- Set Attribute1/LConn1
  Set Attribute1/RConn1 -- Path Combiner/LConn2

== system final_test2/Red Link1 ==
  N-Server : simeventsserver1/N-Server  SystemSampleTime=-1  NumberOfServers=2  ServiceTimeFrom=Dialog  ServiceTime=0.001  AttributeName=ServiceTime  PriorityServiceCompletion=500  EnableTOPort=off  StatNumberDeparted=Off  StatNumberInBlock=Off  StatPendingEntity=Off  StatNumberPending=Off  StatAverageWait=Off  StatUtilization=Off  StatNumberTimedout=Off
  Output Switch : simeventsrouting1/Output Switch  SystemSampleTime=-1  NumberOutputPorts=2  SwitchingCriterion=From attribute  InitialSeed=34567  AttributeName=port  InitialConditionsOpt=off  InitialConditions=1  EntityBufferOpt=off  SpecifyEventPriority=off  PriorityOutputSwitchSelectPort=4100  TimeoutPortOpt=off  StatNumberDeparted=Off  StatNumberTimedOut=Off  StatPendingEntity=Off  StatLastDeparturePort=Off  EvaluatedNumPorts=2
  Path Combiner : simeventsrouting1/Path Combiner  SystemSampleTime=-1  NumberInputPorts=2  InputPortPrecedence=IN1 port  InitialSeed=45675  SpecifyEventPriority=off  PriorityPathCombinerPortPrecedenceSelection=4100  StatNumberDeparted=Off  StatLastArrivalPort=Off  EvaluatedNumPorts=2
  Set Attribute : simeventsattributes2/Set Attribute  SystemSampleTime=-1  AttributeFrom=Dialog  AttributeName=port  AttributeTreatAsVector=1  AttributeValue=1  AttributeCreate=on  StatNumberDeparted=Off  EvaluatedAttributeValue={1}
  Set Attribute1 : simeventsattributes2/Set Attribute  SystemSampleTime=-1  AttributeFrom=Dialog  AttributeName=port  AttributeTreatAsVector=1  AttributeValue=2  AttributeCreate=on  StatNumberDeparted=Off  EvaluatedAttributeValue={2}
  Input1 : PMIOPort  Port=1  Side=Left
  Output1 : PMIOPort  Port=2  Side=Right
  Input2 : PMIOPort  Port=3  Side=Right
  Output2 : PMIOPort  Port=4  Side=Left
  connections:
  Set Attribute1/RConn1 -- Path Combiner/LConn2
  Input2/RConn1 -- Set Attribute1/LConn1
  Set Attribute/RConn1 -- Path Combiner/LConn1
  Input1/RConn1 -- Set Attribute/LConn1
  Output Switch/RConn2 -- Output2/RConn1
  Output Switch/RConn1 -- Output1/RConn1
  N-Server/RConn1 -- Output Switch/LConn1
  Path Combiner/RConn1 -- N-Server/LConn1

== system final_test2/Red Link2 ==
  N-Server : simeventsserver1/N-Server  SystemSampleTime=-1  NumberOfServers=2  ServiceTimeFrom=Dialog  ServiceTime=0.001  AttributeName=ServiceTime  PriorityServiceCompletion=500  EnableTOPort=off  StatNumberDeparted=Off  StatNumberInBlock=Off  StatPendingEntity=Off  StatNumberPending=Off  StatAverageWait=Off  StatUtilization=Off  StatNumberTimedout=Off
  Output Switch : simeventsrouting1/Output Switch  SystemSampleTime=-1  NumberOutputPorts=2  SwitchingCriterion=From attribute  InitialSeed=34567  AttributeName=port  InitialConditionsOpt=off  InitialConditions=1  EntityBufferOpt=off  SpecifyEventPriority=off  PriorityOutputSwitchSelectPort=4100  TimeoutPortOpt=off  StatNumberDeparted=Off  StatNumberTimedOut=Off  StatPendingEntity=Off  StatLastDeparturePort=Off  EvaluatedNumPorts=2
  Path Combiner : simeventsrouting1/Path Combiner  SystemSampleTime=-1  NumberInputPorts=2  InputPortPrecedence=IN1 port  InitialSeed=45675  SpecifyEventPriority=off  PriorityPathCombinerPortPrecedenceSelection=4100  StatNumberDeparted=Off  StatLastArrivalPort=Off  EvaluatedNumPorts=2
  Set Attribute : simeventsattributes2/Set Attribute  SystemSampleTime=-1  AttributeFrom=Dialog  AttributeName=port  AttributeTreatAsVector=1  AttributeValue=1  AttributeCreate=on  StatNumberDeparted=Off  EvaluatedAttributeValue={1}
  Set Attribute1 : simeventsattributes2/Set Attribute  SystemSampleTime=-1  AttributeFrom=Dialog  AttributeName=port  AttributeTreatAsVector=1  AttributeValue=2  AttributeCreate=on  StatNumberDeparted=Off  EvaluatedAttributeValue={2}
  Input1 : PMIOPort  Port=1  Side=Left
  Output1 : PMIOPort  Port=2  Side=Right
  Input2 : PMIOPort  Port=3  Side=Right
  Output2 : PMIOPort  Port=4  Side=Left
  connections:
  Path Combiner/RConn1 -- N-Server/LConn1
  N-Server/RConn1 -- Output Switch/LConn1
  Output Switch/RConn1 -- Output1/RConn1
  Output Switch/RConn2 -- Output2/RConn1
  Input1/RConn1 -- Set Attribute/LConn1
  Set Attribute/RConn1 -- Path Combiner/LConn1
  Input2/RConn1 -- Set Attribute1/LConn1
  Set Attribute1/RConn1 -- Path Combiner/LConn2

== system final_test2/Red Link3 ==
  N-Server : simeventsserver1/N-Server  SystemSampleTime=-1  NumberOfServers=2  ServiceTimeFrom=Dialog  ServiceTime=0.001  AttributeName=ServiceTime  PriorityServiceCompletion=500  EnableTOPort=off  StatNumberDeparted=Off  StatNumberInBlock=Off  StatPendingEntity=Off  StatNumberPending=Off  StatAverageWait=Off  StatUtilization=Off  StatNumberTimedout=Off
  Output Switch : simeventsrouting1/Output Switch  SystemSampleTime=-1  NumberOutputPorts=2  SwitchingCriterion=From attribute  InitialSeed=34567  AttributeName=port  InitialConditionsOpt=off  InitialConditions=1  EntityBufferOpt=off  SpecifyEventPriority=off  PriorityOutputSwitchSelectPort=4100  TimeoutPortOpt=off  StatNumberDeparted=Off  StatNumberTimedOut=Off  StatPendingEntity=Off  StatLastDeparturePort=Off  EvaluatedNumPorts=2
  Path Combiner : simeventsrouting1/Path Combiner  SystemSampleTime=-1  NumberInputPorts=2  InputPortPrecedence=IN1 port  InitialSeed=45675  SpecifyEventPriority=off  PriorityPathCombinerPortPrecedenceSelection=4100  StatNumberDeparted=Off  StatLastArrivalPort=Off  EvaluatedNumPorts=2
  Set Attribute : simeventsattributes2/Set Attribute  SystemSampleTime=-1  AttributeFrom=Dialog  AttributeName=port  AttributeTreatAsVector=1  AttributeValue=1  AttributeCreate=on  StatNumberDeparted=Off  EvaluatedAttributeValue={1}
  Set Attribute1 : simeventsattributes2/Set Attribute  SystemSampleTime=-1  AttributeFrom=Dialog  AttributeName=port  AttributeTreatAsVector=1  AttributeValue=2  AttributeCreate=on  StatNumberDeparted=Off  EvaluatedAttributeValue={2}
  Input1 : PMIOPort  Port=1  Side=Left
  Output1 : PMIOPort  Port=2  Side=Right
  Input2 : PMIOPort  Port=3  Side=Right
  Output2 : PMIOPort  Port=4  Side=Left
  connections:
  Set Attribute1/RConn1 -- Path Combiner/LConn2
  Input2/RConn1 -- Set Attribute1/LConn1
  Set Attribute/RConn1 -- Path Combiner/LConn1
  Input1/RConn1 -- Set Attribute/LConn1
  Output Switch/RConn2 -- Output2/RConn1
  Output Switch/RConn1 -- Output1/RConn1
  N-Server/RConn1 -- Output Switch/LConn1
  Path Combiner/RConn1 -- N-Server/LConn1

== system final_test2/Red Link4 ==
  N-Server : simeventsserver1/N-Server  SystemSampleTime=-1  NumberOfServers=2  ServiceTimeFrom=Dialog  ServiceTime=0.001  AttributeName=ServiceTime  PriorityServiceCompletion=500  EnableTOPort=off  StatNumberDeparted=Off  StatNumberInBlock=Off  StatPendingEntity=Off  StatNumberPending=Off  StatAverageWait=Off  StatUtilization=Off  StatNumberTimedout=Off
  Output Switch : simeventsrouting1/Output Switch  SystemSampleTime=-1  NumberOutputPorts=2  SwitchingCriterion=From attribute  InitialSeed=34567  AttributeName=port  InitialConditionsOpt=off  InitialConditions=1  EntityBufferOpt=off  SpecifyEventPriority=off  PriorityOutputSwitchSelectPort=4100  TimeoutPortOpt=off  StatNumberDeparted=Off  StatNumberTimedOut=Off  StatPendingEntity=Off  StatLastDeparturePort=Off  EvaluatedNumPorts=2
  Path Combiner : simeventsrouting1/Path Combiner  SystemSampleTime=-1  NumberInputPorts=2  InputPortPrecedence=IN1 port  InitialSeed=45675  SpecifyEventPriority=off  PriorityPathCombinerPortPrecedenceSelection=4100  StatNumberDeparted=Off  StatLastArrivalPort=Off  EvaluatedNumPorts=2
  Set Attribute : simeventsattributes2/Set Attribute  SystemSampleTime=-1  AttributeFrom=Dialog  AttributeName=port  AttributeTreatAsVector=1  AttributeValue=1  AttributeCreate=on  StatNumberDeparted=Off  EvaluatedAttributeValue={1}
  Set Attribute1 : simeventsattributes2/Set Attribute  SystemSampleTime=-1  AttributeFrom=Dialog  AttributeName=port  AttributeTreatAsVector=1  AttributeValue=2  AttributeCreate=on  StatNumberDeparted=Off  EvaluatedAttributeValue={2}
  Input1 : PMIOPort  Port=1  Side=Left
  Output1 : PMIOPort  Port=2  Side=Right
  Input2 : PMIOPort  Port=3  Side=Right
  Output2 : PMIOPort  Port=4  Side=Left
  connections:
  Path Combiner/RConn1 -- N-Server/LConn1
  N-Server/RConn1 -- Output Switch/LConn1
  Output Switch/RConn1 -- Output1/RConn1
  Output Switch/RConn2 -- Output2/RConn1
  Input1/RConn1 -- Set Attribute/LConn1
  Set Attribute/RConn1 -- Path Combiner/LConn1
  Input2/RConn1 -- Set Attribute1/LConn1
  Set Attribute1/RConn1 -- Path Combiner/LConn2
